simulink model "reflow_oven_simulation"  (R2025b)
settings: Solver=VariableStepAuto  StartTime=0.0  StopTime=245  RelTol=1e-3
libraries: SignalEditorBlockLib x2, slpidlib x1
settings Model: Creator=stevenketiah  LastModifiedBy=stevenketiah

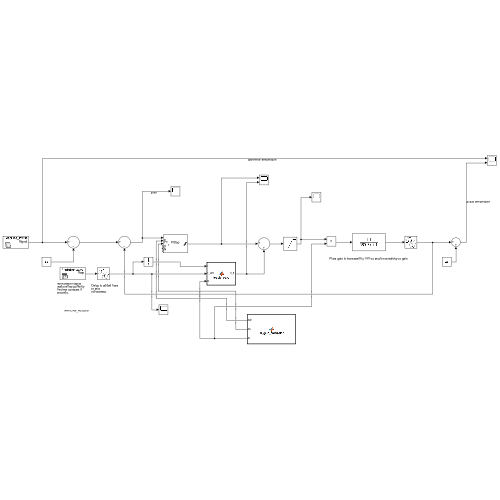
[thumbnail: Simulink's stored preview of the top-level diagram]
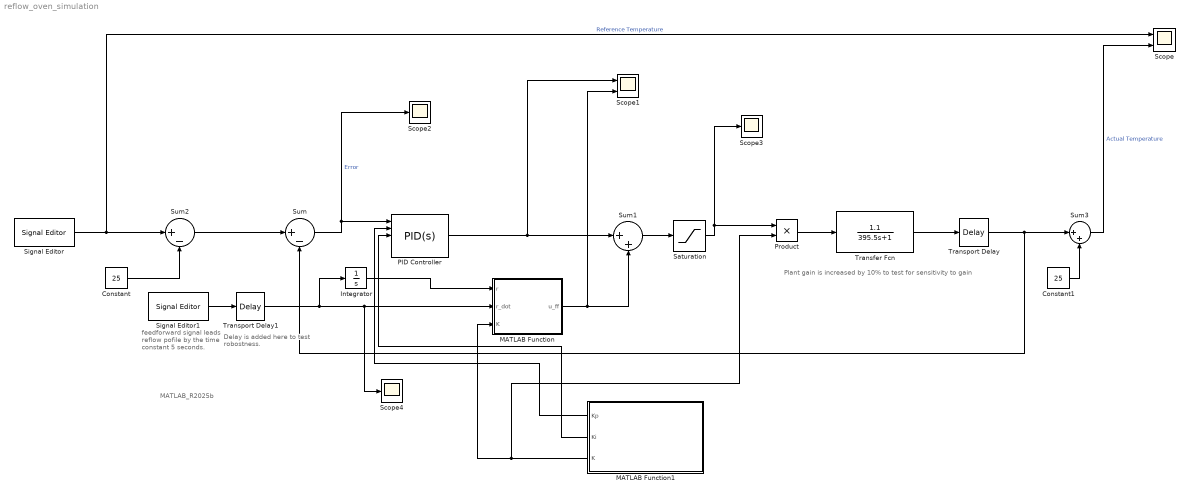
== system reflow_oven_simulation ==
  note: MATLAB_R2025b
  note: Plant gain is increased by 10% to test for sensitivity to gain
  note: feedforward signal leads reflow pofile by the time constant 5 seconds.
  note: Delay is added here to test
      | robostness.
  Constant : Constant  Value=25
  Constant1 : Constant  Value=25
  Integrator : Integrator
  MATLAB Function : MATLAB Function  TreatAsAtomicUnit=on
  MATLAB Function1 : MATLAB Function  TreatAsAtomicUnit=on
  PID Controller : slpidlib/PID Controller  Controller=PID  Form=Parallel  TimeDomain=Continuous-time  UseExternalTs=off  SampleTime=-1  IntegratorMethod=Forward Euler  FilterMethod=Forward Euler  ControllerParametersSource=external  P=0.0101  I=0.0000201  UseKiTs=on  D=0  UseExternalDerivativeSource=off  N=100  UseFilter=on  TunerSelectOption=Transfer Function Based (PID Tuner App)  InitialConditionSource=internal  InitialConditionForIntegrator=0  InitialConditionForFilter=0  DifferentiatorICPrevScaledInput=0  ExternalReset=none  TrackingMode=off  Kt=1  LimitOutput=on  SatLimitsSource=internal  UpperSaturationLimit=1  LowerSaturationLimit=-1  LinearizeAsGain=on  AntiWindupMode=clamping  Kb=1  LimitIntegrator=off  UpperIntegratorSaturationLimit=inf  LowerIntegratorSaturationLimit=-inf  POutMin=[]  POutMax=[]  IOutMin=[]  IOutMax=[]  DOutMin=[]  DOutMax=[]  NOutMin=[]  NOutMax=[]  SumOutMin=[]  SumOutMax=[]  SaturationOutMin=[]  SaturationOutMax=[]  PParamMin=[]  PParamMax=[]  IParamMin=[]  IParamMax=[]  DParamMin=[]  DParamMax=[]  NParamMin=[]  NParamMax=[]  KbParamMin=[]  KbParamMax=[]  KtParamMin=[]  KtParamMax=[]  KbOutMin=[]  KbOutMax=[]  KtOutMin=[]  KtOutMax=[]  IntegratorOutMin=[]  IntegratorOutMax=[]  FilterOutMin=[]  FilterOutMax=[]  SumI1OutMin=[]  SumI1OutMax=[]  SumI2OutMin=[]  SumI2OutMax=[]  SumI3OutMin=[]  SumI3OutMax=[]  SumI4OutMin=[]  SumI4OutMax=[]  SumDOutMin=[]  SumDOutMax=[]  DifferentiatorOutMin=[]  DifferentiatorOutMax=[]  FilterDiffOutCoefMin=[]  FilterDiffOutCoefMax=[]  ReciprocalOutMin=[]  ReciprocalOutMax=[]  SumDenOutMin=[]  SumDenOutMax=[]  SumNumOutMin=[]  SumNumOutMax=[]  DivideOutMin=[]  DivideOutMax=[]  UdiffTsProdOutMin=[]  UdiffTsProdOutMax=[]  NTsProdOutMin=[]  NTsProdOutMax=[]  UintegralTsProdOutMin=[]  UintegralTsProdOutMax=[]  UngainTsProdOutMin=[]  UngainTsProdOutMax=[]  ClampingZeroOutDataTypeStr=Inherit: Inherit via back propagation  ClampingZeroOutMin=[]  ClampingZeroOutMax=[]  FilterDenConstantOutDataTypeStr=Inherit: Inherit via back propagation  FilterDenConstantOutMin=[]  FilterDenConstantOutMax=[]  PCopyOutDataTypeStr=Inherit: Inherit via back propagation  PCopyOutMin=[]  PCopyOutMax=[]  NCopyOutDataTypeStr=Inherit: Inherit via back propagation  NCopyOutMin=[]  NCopyOutMax=[]  IntegratorContinuousStateAttributes=''  IntegratorStateMustResolveToSignalObject=off  IntegratorRTWStateStorageClass=Auto  FilterContinuousStateAttributes=''  FilterStateMustResolveToSignalObject=off  FilterRTWStateStorageClass=Auto  ParallelPVariant=ExternalParameters  IdealPVariant=Disabled  IVariant=ExternalParameters  DVariant=ExternalParameters  IntegratorVariant=Continuous  SatVariant=Enabled  AWVariant=ContClampingParallel  PCopyVariant=Disabled  TRVariant=Disabled  FdbkBlocksVariant=Forward  IdealPFdbkVariant=Disabled  SatFdbkVariant=Disabled  DerivativeFilterVariant=ContFilter  NVariant=ExternalParameters  NCopyVariant=Disabled  FilterICVariant=InternalICsFilter  IntegratorICVariant=InternalICs  ExternalResetVariant=Disabled  TRSumVariant=Passthrough  SumFdbkVariant=Disabled  SumVariant=Sum_PID  TsampFilterVariant=InternalTs  TsampNgainVariant=Passthrough  TsampIntegralVariant=Disabled_SignalSpec  ExternalSaturationOutDataTypeStr=Inherit: Same as second input  DerivativeSourceVariant=ErrorSignal  PreIntVariant=InternalPreInt
  Product : Product
  Saturation : Saturate  UpperLimit=1  LowerLimit=0
  Scope : Scope  NumInputPorts=2
      settings: Title=Temperature  ActiveDisplayYMinimum=3.2738462310569219  ActiveDisplayYMaximum=340.65948301067738
  Scope1 : Scope  NumInputPorts=2
      settings: ActiveDisplayYMinimum=-0.23135619596375029  ActiveDisplayYMaximum=1.2219963676191665
  Scope2 : Scope
      settings: Title=Error  ActiveDisplayYMinimum=-5.5170999680462094  ActiveDisplayYMaximum=3.716845179250146  DataLoggingVariableName=ScopeData2
  Scope3 : Scope
      settings: ActiveDisplayYMinimum=0.15356234029583077  ActiveDisplayYMaximum=1.0677980340249431  DataLoggingVariableName=ScopeData3
  Scope4 : Scope
      settings: ActiveDisplayYMinimum=-0.20833333333333329  ActiveDisplayYMaximum=1.875  DataLoggingVariableName=ScopeData4
  Signal Editor : SignalEditorBlockLib/Signal Editor  FileName=reflow_profile.mat  ActiveScenario=LeadFree_Profile  ActiveSignal=Signal  IsBus=off  OutputBusObjectStr=Bus: BusObject  SampleTime=0  ZeroCross=off  OutputAfterFinalValue=Setting to zero  Unit=inherit  PreserveSignalName=on  ApplySigPropsToAllScenarios=on  ApplySigPropsToAllSignals=off  SignalPropertySource=Dialog parameters
  Signal Editor1 : SignalEditorBlockLib/Signal Editor  FileName=reflo_profile_without_delay.mat  ActiveScenario=ProfileDerivative  ActiveSignal=Step  IsBus=off  OutputBusObjectStr=Bus: BusObject  SampleTime=0  ZeroCross=off  OutputAfterFinalValue=Setting to zero  Unit=inherit  PreserveSignalName=on  ApplySigPropsToAllScenarios=on  ApplySigPropsToAllSignals=off  SignalPropertySource=Dialog parameters
  Sum : Sum  Inputs=|+-
  Sum1 : Sum  Inputs=|++
  Sum2 : Sum  Inputs=|+-
  Sum3 : Sum  Inputs=|++
  Transfer Fcn : TransferFcn  Numerator=[1.1]  Denominator=[395.5 1]
  Transport Delay : TransportDelay  DelayTime=5
  Transport Delay1 : TransportDelay  DelayTime=2
  wires:
  Sum/1 -> Scope2/1, PID Controller/1  "Error"
  PID Controller/1 -> Scope1/1, Sum1/1
  Sum1/1 -> Saturation/1
  MATLAB Function/1(u_ff) -> Scope1/2, Sum1/2
  Transport Delay/1 -> Sum/2, Sum3/1
  Sum2/1 -> Sum/1
  Saturation/1 -> Product/1, Scope3/1
  Constant/1 -> Sum2/2
  Sum3/1 -> Scope/2  "Actual Temperature"
  Constant1/1 -> Sum3/2
  Signal Editor/1 -> Scope/1, Sum2/1  "Reference Temperature"
  Integrator/1 -> MATLAB Function/1(r)
  MATLAB Function1/3(K) -> Product/2, MATLAB Function/3(K)
  MATLAB Function1/1(Kp) -> PID Controller/2
  MATLAB Function1/2(Ki) -> PID Controller/3
  Product/1 -> Transfer Fcn/1
  Transfer Fcn/1 -> Transport Delay/1
  Signal Editor1/1 -> Transport Delay1/1
  Transport Delay1/1 -> Integrator/1, MATLAB Function/2(r_dot), Scope4/1

== matlab function reflow_oven_simulation/MATLAB Function1 ==
  data: Kp output; Ki output; K output
function [Kp, Ki, K] = pi_gain_calculator()
    % Tuning parameters (adjust these)
    theta = 5;      % Dead time estimate (seconds) - measure from your step tests
    tau_c = 1*theta;     % Desired closed-loop time constant (seconds) - tune for speed vs robustness
    tau = 395.5;

   
    K = 666.49;
    
    % SIMC tuning rules
    Kp = 1 * tau / (K * (tau_c + theta));
    Ki =  1  / (K * (tau_c + theta));

end

== matlab function reflow_oven_simulation/MATLAB Function ==
  data: r input; u_ff output; r_dot input; K input
function u_ff = feedforward(r,  r_dot, K)
    tau = 395.5;

    u_ff = (tau * r_dot + r) / K;
end
